simulink model "UseFmu_Seperator"  (R2020b)
settings: Solver=FixedStepDiscrete  StartTime=0.0  StopTime=Inf  FixedStep=0.010  RelTol=1e-3
settings Model: Creator=kaebi  LastModifiedBy=kaebi
settings OptimizationCC: DefaultParameterBehavior=Inlined  LocalBlockOutputs=off
settings RTWCC: Description=TwinCAT GRT Target  SystemTargetFile=TwinCatGrt.tlc  GenCodeOnly=on  TemplateMakefile=tcgrt_msbuild.tmf  TargetLang=C++
settings STFCustomTargetCC: TargetLangStandard=C++03 (ISO)  ConcurrentExecutionCompliant=off  CombineOutputUpdateFcns=on  CodeInterfacePackaging=Reusable function  GRTInterface=off  GenerateAllocFcn=on  SystemTargetFile=TwinCatGrt.tlc
settings GRTTargetCC: TargetLangStandard=C++03 (ISO)  ParMdlRefBuildCompliant=off  CompOptLevelCompliant=off  ConcurrentExecutionCompliant=off  MatFileLogging=off  CodeInterfacePackaging=Reusable function  GenerateAllocFcn=on  UseToolchainInfoCompliant=off  ExtModeMexFile=TcExtModeClient

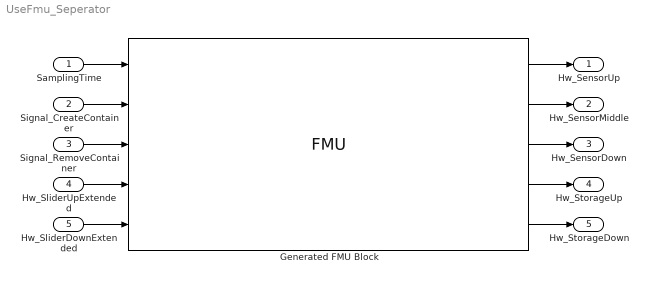
== system UseFmu_Seperator ==
  SamplingTime : Inport
  Signal_CreateContainer : Inport  Port=2
  Signal_RemoveContainer : Inport  Port=3
  Hw_SliderUpExtended : Inport  Port=4
  Hw_SliderDownExtended : Inport  Port=5
  Generated FMU Block : FMU  FMUName=CreateFmu_Seperator  FMUMode=CoSimulation
      mask Type: CreateFmu_Seperator [Co-Simulation, v2.0]
      mask Display:
      | if (exist([Simulink.fileGenControl('get','CacheFolder') '\slprj\_fmu\9f468976759720a38a9808d7ed60361a\CreateFmu_Seperator\model.png'],'file'))
      |     image([Simulink.fileGenControl('get','CacheFolder') '\slprj\_fmu\9f468976759720a38a9808d7ed60361a\CreateFmu_Seperator\model.png']);
      | else
      |     disp('CreateFmu_Seperator');
      | end
      | port_label('output',1,'Hw_SensorUp');
      | port_label('output',2,'HW_SensorMiddle');
      | port_label('output',3,'HW_SensorDown');
      | port_label('output',4,'Signal_StorageUp');
      | port_label('output',5,'Signal_StorageDown');
      | port_label('input',1,'SamplingTime');
      | port_label('input',2,'Signal_CreateContainer');
      | port_label('input',3,'Signal_RemoveContainer');
      | port_label('input',4,'Hw_SliderUpExtended');
      | port_label('input',5,'HW_SliderDownExtended');
  Hw_SensorUp : Outport
  Hw_SensorMiddle : Outport  Port=2
  Hw_SensorDown : Outport  Port=3
  Hw_StorageUp : Outport  Port=4
  Hw_StorageDown : Outport  Port=5
  wires:
  Hw_SliderUpExtended/1 -> Generated FMU Block/4
  Signal_RemoveContainer/1 -> Generated FMU Block/3
  Signal_CreateContainer/1 -> Generated FMU Block/2
  Generated FMU Block/1 -> Hw_SensorUp/1
  Generated FMU Block/4 -> Hw_StorageUp/1
  Generated FMU Block/3 -> Hw_SensorDown/1
  Generated FMU Block/2 -> Hw_SensorMiddle/1
  SamplingTime/1 -> Generated FMU Block/1
  Hw_SliderDownExtended/1 -> Generated FMU Block/5
  Generated FMU Block/5 -> Hw_StorageDown/1
